simulink model "HW2_Exercise2_Step"  (R2017a)
settings: Solver=ode5  StartTime=0.0  StopTime=1  FixedStep=0.01  RelTol=1e-3
undefined symbols (not defined in the file): k_d, k_i, k_p, m
settings Model: Creator=Alfred  LastModifiedBy=Alfred

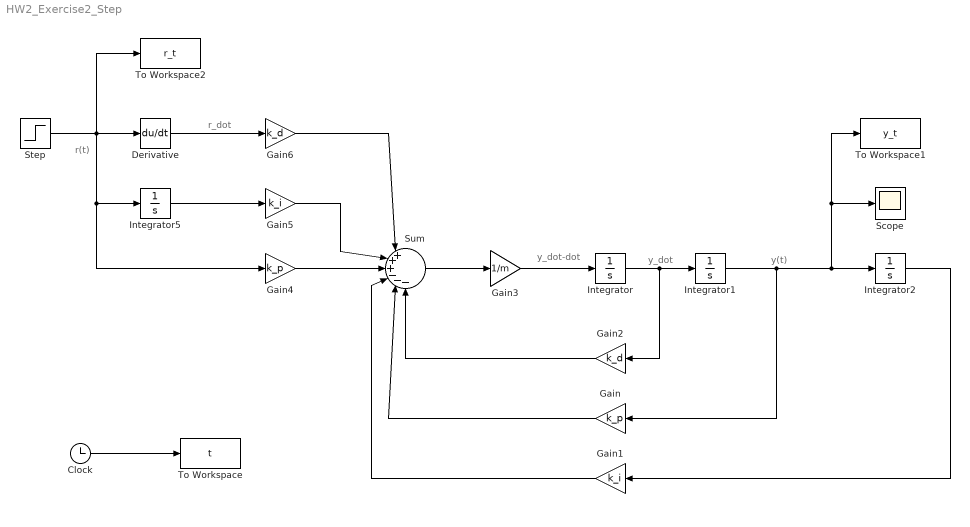
== system HW2_Exercise2_Step ==
  note: r_dot
  note: r(t)
  note: y(t)
  note: y_dot
  note: y_dot-dot
  Clock : Clock
  Derivative : Derivative
  Gain : Gain  Gain=k_p
  Gain1 : Gain  Gain=k_i
  Gain2 : Gain  Gain=k_d
  Gain3 : Gain  Gain=1/m
  Gain4 : Gain  Gain=k_p
  Gain5 : Gain  Gain=k_i
  Gain6 : Gain  Gain=k_d
  Integrator{,1..2,5} (4 alike) : Integrator
  Scope : Scope
  Step : Step  Time=0.01  SampleTime=0
  Sum : Sum  Inputs=|+++---
  To Workspace : ToWorkspace  VariableName=t  SampleTime=-1
      settings: Save2DSignal=2-D array (concatenate along first dimension)
  To Workspace1 : ToWorkspace  VariableName=y_t  SampleTime=-1
      settings: Save2DSignal=2-D array (concatenate along first dimension)
  To Workspace2 : ToWorkspace  VariableName=r_t  SampleTime=-1
      settings: Save2DSignal=2-D array (concatenate along first dimension)
  wires:
  Gain3/1 -> Integrator/1
  Sum/1 -> Gain3/1
  Integrator/1 -> Gain2/1, Integrator1/1
  Integrator1/1 -> Gain/1, To Workspace1/1, Scope/1, Integrator2/1
  Integrator2/1 -> Gain1/1
  Clock/1 -> To Workspace/1
  Gain2/1 -> Sum/6
  Gain/1 -> Sum/5
  Gain1/1 -> Sum/4
  Step/1 -> To Workspace2/1, Integrator5/1, Gain4/1, Derivative/1
  Integrator5/1 -> Gain5/1
  Gain5/1 -> Sum/2
  Derivative/1 -> Gain6/1
  Gain6/1 -> Sum/1
  Gain4/1 -> Sum/3
